simulink model "System_R1"  (R2018b)
settings: Solver=VariableStepAuto  StartTime=0.0  StopTime=5  RelTol=1e-3
libraries: dspsrcs4 x1
settings Model: Creator=Whtest  LastModifiedBy=Whtest

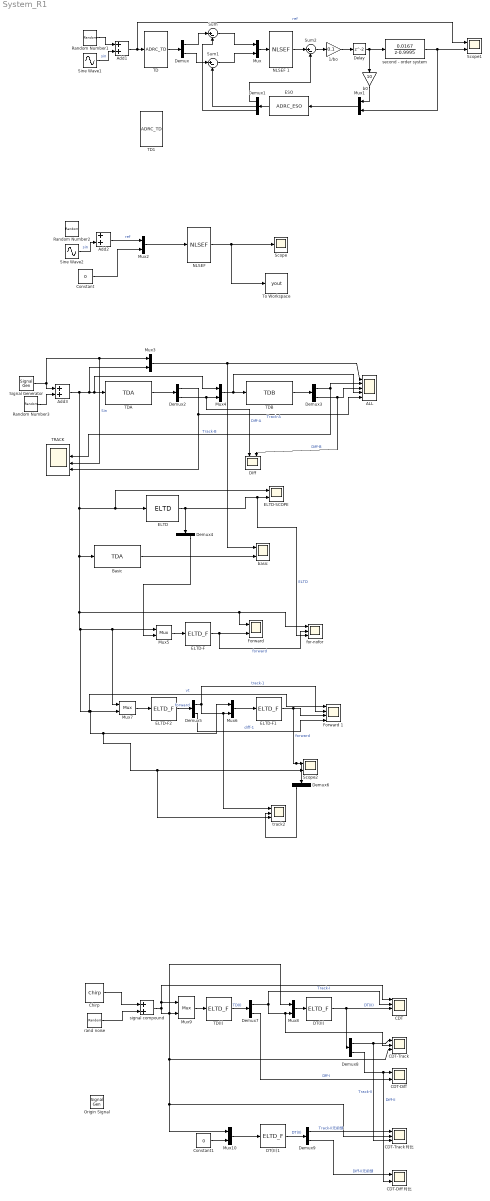
== system System_R1 ==
  "1/bo " : Gain  Gain=0.1
  "ALL " : Scope  NumInputPorts=5
  Add1 : Sum
  Add2 : Sum
  Add3 : Sum
  Basic : S-Function  FunctionName=TDA  Parameters=20,1e2  SFunctionDeploymentMode=off  EnableBusSupport=off
  CDT : Scope  NumInputPorts=4
  CDT-Diff : Scope  NumInputPorts=2
  CDT-Diff对比 : Scope  NumInputPorts=2
  CDT-Track : Scope  NumInputPorts=3
  "CDT-Track对比 " : Scope  NumInputPorts=3
  Chirp : dspsrcs4/Chirp  sweep=Linear  mode=Unidirectional  f0=1  f1=5  t1=5  Tsweep=5  phase=1.5*pi  Ts=0.001  spf=1  datatype=Double  OutputFrames=off
      settings: SourceProductName=DSP System Toolbox
  Constant : Constant  Value=0  SampleTime=1e-3
  Constant1 : Constant  Value=0
  "DIff " : Scope  NumInputPorts=2
  DT(II) : S-Function  FunctionName=ELTD_F  Parameters=2.2,2.8,30,40  SFunctionDeploymentMode=off  EnableBusSupport=off
  DT(II)1 : S-Function  FunctionName=ELTD_F  Parameters=2.2,2.8,30,40  SFunctionDeploymentMode=off  EnableBusSupport=off
  Delay : Delay
  Demux{,2..9} (9 alike) : Demux  Outputs=2
  Demux1 : Demux  Outputs=3
  "ELTD " : S-Function  FunctionName=ELTD  Parameters=3,3,30  SFunctionDeploymentMode=off  EnableBusSupport=off
  ELTD-F : S-Function  FunctionName=ELTD_F  Parameters=3,3,30,1  SFunctionDeploymentMode=off  EnableBusSupport=off
  ELTD-F1 : S-Function  FunctionName=ELTD_F  Parameters=2.2,2.8,150,40  SFunctionDeploymentMode=off  EnableBusSupport=off
  ELTD-F2 : S-Function  FunctionName=ELTD_F  Parameters=2.2,1.3,15,5  SFunctionDeploymentMode=off  EnableBusSupport=off
  "ELTD-SCOPE " : Scope  NumInputPorts=2
  ESO : S-Function  FunctionName=ADRC_ESO  Parameters=1 1 1 1 1 1  SFunctionDeploymentMode=off  EnableBusSupport=off
  "Forward " : Scope  NumInputPorts=2
  Forward 1 : Scope  NumInputPorts=4
  Mux{,1..10} (11 alike) : Mux  Inputs=2
      Mux5 settings: DisplayOption=signals
      Mux7 settings: DisplayOption=signals
      Mux9 settings: DisplayOption=signals
  "NLSEF " : S-Function  FunctionName=NLSEF  Parameters=0.5,0.5,1,0.5,0.5,1  SFunctionDeploymentMode=off  EnableBusSupport=off
  NLSEF 1 : S-Function  FunctionName=NLSEF  Parameters=0.5,0.5,2,0.5,0.5,2  SFunctionDeploymentMode=off  EnableBusSupport=off
  Origin Signal : SignalGenerator  Frequency=6.18  Units=rad/sec
  Random Number1 : RandomNumber  Variance=0.1  SampleTime=0.001
  Random Number2 : RandomNumber  Variance=0.1  SampleTime=0.001
  Random Number3 : RandomNumber  Variance=0.04  SampleTime=0.001
  Scope : Scope
  Scope1 : Scope  NumInputPorts=2
  Scope2 : Scope  NumInputPorts=2
  Signal Generator : SignalGenerator  WaveForm=square  Amplitude=10000  Frequency=5
  Sine Wave1 : Sin  Amplitude=5  Frequency=6.28  SampleTime=1e-3
  Sine Wave2 : Sin  Frequency=6.28  SampleTime=1e-3
  Sum : Sum  Inputs=|+-
  Sum1 : Sum  Inputs=|+-
  Sum2 : Sum  Inputs=|+-
  TD : S-Function  FunctionName=ADRC_TD  Parameters=1e-2,5e6  SFunctionDeploymentMode=off  EnableBusSupport=off
  TD(I) : S-Function  FunctionName=ELTD_F  Parameters=2.2,1.3,30,15  SFunctionDeploymentMode=off  EnableBusSupport=off
  TD1 : S-Function  FunctionName=ADRC_TD  Parameters=1e-2,5e6  SFunctionDeploymentMode=off  EnableBusSupport=off
  TDA : S-Function  FunctionName=TDA  Parameters=20,1e3  SFunctionDeploymentMode=off  EnableBusSupport=off
  "TDB " : S-Function  FunctionName=TDB  Parameters=20,1e4,0.02  SFunctionDeploymentMode=off  EnableBusSupport=off
  "TRACK " : Scope  NumInputPorts=4
  To Workspace : ToWorkspace  VariableName=yout  SampleTime=-1
      settings: Save2DSignal=2-D array (concatenate along first dimension)
  b0 : Gain  Gain=10
  "basic " : Scope  NumInputPorts=2
  "for-nofor " : Scope  NumInputPorts=3
  rand noise : RandomNumber  Variance=0.01  SampleTime=0.001
  second - order system : DiscreteTransferFcn  Numerator="[0    0.0167]"  Denominator="[1.0000   -0.9995]"
  signal compound : Sum
  "track2 " : Scope  NumInputPorts=3
  wires:
  Random Number1/1 -> Add1/1
  Sine Wave1/1 -> Add1/2  "sin"
  Demux/1 -> Sum/1
  Demux/2 -> Sum1/1
  Sum/1 -> Mux/1
  Sum1/1 -> Mux/2
  Mux/1 -> NLSEF 1/1
  Add1/1 -> Scope1/1, TD/1  "ref"
  TD/1 -> Demux/1
  ESO/1 -> Demux1/1
  NLSEF 1/1 -> Sum2/1
  Sum2/1 -> "1/bo "/1
  "1/bo "/1 -> Delay/1
  Delay/1 -> second - order system/1, b0/1
  second - order system/1 -> Scope1/2, Mux1/2
  Mux1/1 -> ESO/1
  b0/1 -> Mux1/1
  Demux1/1 -> Sum2/2
  Demux1/2 -> Sum1/2
  Demux1/3 -> Sum/2
  Sine Wave2/1 -> Add2/2  "sin"
  Add2/1 -> Mux2/1  "ref"
  "NLSEF "/1 -> To Workspace/1, Scope/1
  Constant/1 -> Mux2/2
  Mux2/1 -> "NLSEF "/1
  TDA/1 -> Demux2/1
  Mux4/1 -> "ALL "/4, "TDB "/1
  "TDB "/1 -> Demux3/1
  Add3/1 -> "ELTD-SCOPE "/1, "ELTD "/1, "for-nofor "/1, "Forward "/1, Forward 1/1, "track2 "/3, Scope2/2, Mux6/1, Mux7/2, Mux7/1, Mux5/1, Basic/1, Mux4/1, TDA/1, Mux3/2  "vt"
  Mux3/1 -> "basic "/1, "ALL "/1
  Signal Generator/1 -> Mux3/1, "TRACK "/3, Add3/1  "Sin"
  Demux3/1 -> "ALL "/2, "TRACK "/2  "Track-B"
  Demux3/2 -> "DIff "/2, "ALL "/3  "Diff-B"
  Demux2/2 -> "DIff "/1, Mux4/2  "Diff-A"
  Demux2/1 -> "TRACK "/4, "ALL "/5  "Track-A"
  "ELTD "/1 -> "for-nofor "/3, "ELTD-SCOPE "/2, Demux4/1  "ELTD"
  Basic/1 -> "basic "/2
  Mux5/1 -> ELTD-F/1
  ELTD-F/1 -> "for-nofor "/2, "Forward "/2  "forward"
  Demux4/2 -> Mux5/2
  ELTD-F2/1 -> Demux5/1  "forward"
  Mux7/1 -> ELTD-F2/1
  Mux6/1 -> ELTD-F1/1
  ELTD-F1/1 -> Demux6/1, Scope2/1, Forward 1/3  "forward"
  Demux5/1 -> "track2 "/1, Mux6/2, Forward 1/2  "track-1"
  Random Number3/1 -> Add3/2
  Demux5/2 -> Forward 1/4  "diff-1"
  Demux6/1 -> "track2 "/2
  Demux7/1 -> CDT/2, CDT-Track/2, Mux8/2  "Track-I"
  Mux8/1 -> DT(II)/1
  TD(I)/1 -> Demux7/1  "TD(I)"
  DT(II)/1 -> Demux8/1, CDT/3  "DT(II)"
  rand noise/1 -> signal compound/2
  Mux9/1 -> TD(I)/1
  signal compound/1 -> CDT/1, Mux9/1, CDT-Track/3, "CDT-Track对比 "/2, Mux10/1, Mux8/1, Mux9/2
  Demux7/2 -> CDT-Diff/2  "Dff-I"
  Demux8/2 -> CDT-Diff对比/2, CDT-Diff/1  "Diff-II"
  Demux8/1 -> "CDT-Track对比 "/3, CDT-Track/1  "Track-II"
  DT(II)1/1 -> Demux9/1  "DT(II)"
  Demux9/1 -> "CDT-Track对比 "/1  "Track-II无前馈"
  Demux9/2 -> CDT-Diff对比/1  "Diff-II无前馈"
  Mux10/1 -> DT(II)1/1
  Constant1/1 -> Mux10/2
  Chirp/1 -> signal compound/1
